simulink library "Lib_Turbo_Nozzle_TMATS"  (R2019b)
settings: Solver=ode45  StartTime=0.0  StopTime=10.0  RelTol=1e-3  EnableMultiTasking=on
undefined symbols (not defined in the file): stripchar_TMATS
libraries: Lib_Solve_DataOut_TMATS x1
Description:
  | Thomas Modules
settings Model: Creator=jwchapm2  LastModifiedBy=bhisma
settings DataIOCC: LimitDataPoints=on  SaveFormat=Array  ReturnWorkspaceOutputs=off
settings OptimizationCC: ExpressionDepthLimit=2147483647  LifeSpan=inf
settings DebuggingCC: UnderspecifiedInitializationDetection=Classic  MergeDetectMultiDrivingBlocksExec=none  SolverPrmCheckMsg=warning  StateNameClashWarn=warning  SFUnexpectedBacktrackingDiag=warning  SFNoUnconditionalDefaultTransitionDiag=warning  SFExecutionAtInitializationDiag=none  ArithmeticOperatorsInVariantConditions=warning
settings HardwareCC: ProdBitPerPointer=32  ProdBitPerSizeT=32  ProdBitPerPtrDiffT=32  ProdLargestAtomicFloat=None  ProdIntDivRoundTo=Undefined  ProdEndianess=Unspecified  ProdWordSize=32  ProdHWDeviceType=32-bit Generic
settings ModelReferenceCC: PropagateSignalLabelsOutOfModel=off
settings SFSimCC: SimUseLocalCustomCode=off  CustomCodeUndefinedFunction=UseInterfaceOnly
settings RTWCC: RTWUseLocalCustomCode=off
settings CodeAppCC: StateflowObjectComments=on
settings GRTTargetCC: TargetLangStandard=C89/C90 (ANSI)  GeneratePreprocessorConditionals=Disable all
settings ConfigComp: CovMetricSettings=dw  CovHtmlReporting=on  CovSaveCumulativeToWorkspaceVar=on  CovSaveSingleToWorkspaceVar=on  CovExternalEMLEnable=off

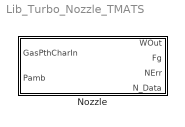
== system Lib_Turbo_Nozzle_TMATS ==
  Nozzle : Subsystem  mask(T-MATS: Nozzle Library Block){SWType_M=Convergent, N_TArea_M=110.7, N_EArea_M=110.7, N_FL_M=0.00, X_N_TtVec2_M=[300 10000], T_N_TGArray_M=[1 1], X_N_PEQPaVec_M=[0 10000], T_N_CdThArray_M=[1 1], T_N_CvArray_M=[1 1], CfgEn_M=off, T_N_CfgArray_M=[1 1], X_N_FARVec_M=[0; 0.0050; 0.0100; 0.0150; 0.0200; 0.0250; 0.0300], T_N_RtArray_M=[0.0686;    0.0686;    0.0686;    0.0686;    0.0686;    0.0686;    0.0686], Y_N_TtVec_M=[300 10000], T_N_MAP_gammaArray_M=[ 1.4 1.4 1.4 1.4 1.4 1.4 1.4; 1.4 1.4 1.4 1.4 1.4 1.4 1.4], iDesign_M=0, WDes_M=100, FVar_M=strcat('iDes_',stripchar_TMATS(gcb),'.bin')}
      mask prompts: SWType_M "SWType_M - Nozzle Type"; N_TArea_M "N_TArea_M - Nozzle Throat Area [in^2]"; N_EArea_M "N_EArea_M - Nozzle Exit Area [in^2], for CD nozzle only"; N_FL_M "N_FL_M - Flow Loss Across Nozzle [%]"; X_N_TtVec2_M "X_N_TtVec2_M - Nozzle Total Temperature Vector (X-axis for TG calc)(ax1)"; T_N_TGArray_M "T_N_TGArray_M - Nozzle Thermal Growth Array (TG = f(Tt))(ax1)"; X_N_PEQPaVec_M "X_N_PEQPaVec_M - Nozzle PE/Pa Vector (X-axis) (bx1)"; T_N_CdThArray_M "T_N_CdThArray_M - Nozzle CdTh Array, Blockage Factor [frac] (CdTh = f(PEQPa)) (bx1)"; T_N_CvArray_M "T_N_CvArray_M - Nozzle Velocity Coefficient Array (Cv = f(PEQPa)) (bx1)"; CfgEn_M "CfgEn_M - Enable Nozzle Thrust Coefficient"; T_N_CfgArray_M "T_N_CfgArray_M - Nozzle Thrust Coefficient Array (Cfg = f(PEQPa)) (bx1)"; X_N_FARVec_M "X_N_FARVec_M - Nozzle Fuel to Air Ratio Vector (X-axis) (cx1)"; T_N_RtArray_M "T_N_RtArray_M - Nozzle Gas Constant, R, Array (R = f(FAR))(cx1)"; Y_N_TtVec_M "Y_N_TtVec_M - Nozzle Total Temperature Vector (Y-axis for Gamma calc)(dx1)"; T_N_MAP_gammaArray_M "T_N_MAP_gammaArray_M - Nozzle Map Gamma Array (Gamma = f(Tt,FAR))(dxc)"; iDesign_M "iDesign_M - Design fork (0 - Enable iDes, 1 - Use iDes Ath, 2 - Use Input Ath)"; WDes_M "WDes_M - Design Flow [pps]"; FVar_M "FVar_M - File name for iDes Variables"
      mask help: This block simulates the performance of a nozzle using basic thermodynamic equations, properties, and table lookups.
      mask init:
      | if iDesign_M == 1
      |     P = load(FVar_M);
      |     N_TArea_M = P(1);
      |     N_EArea_M = P(2);
      | end
      mask Help: web(which('Turbo_TMATS_Noz.html'),'-helpbrowser')
      mask TypeOptions SWType_M: Convergent | Convergent-Divergent
      mask Callback SWType_M:
      | switch get_param(gcb,'iDesign_M')
      |     case ('2')
      |         switch get_param(gcb,'SWType_M')
      |             case ('Convergent')
      |                 MSK_SEC_Enables_Ides_TMATS(int16(1),[3],'G1')
      |             case ('Convergent-Divergent')
      |                 MSK_SEC_Enables_Ides_TMATS(int16(2),[3],'G1')
      |         end
      | end
      mask Callback CfgEn_M:
      | MSK_SEC_Enables_TMATS('CfgEn_M',[11],'en')
      | MSK_SEC_Enables_TMATS('CfgEn_M',[9],'dis')
      mask Callback iDesign_M:
      | switch get_param(gcb,'SWType_M')
      |     case ('Convergent-Divergent')
      |     MSK_SEC_Enables_Ides_TMATS('iDesign_M',[3],'G1')
      | end
      | 
      | MSK_SEC_Enables_Ides_TMATS('iDesign_M',[2],'G1')
      | MSK_SEC_Enables_Ides_TMATS('iDesign_M',[17],'G2')
      | MSK_SEC_Enables_Ides_TMATS('iDesign_M',[18],'G3')
      mask DialogControl ParameterTabVar0 Prompt: General
      mask DialogControl ParameterTabVar01 Prompt: GasProp
      mask DialogControl ParameterTabVar012 Prompt: iDesign

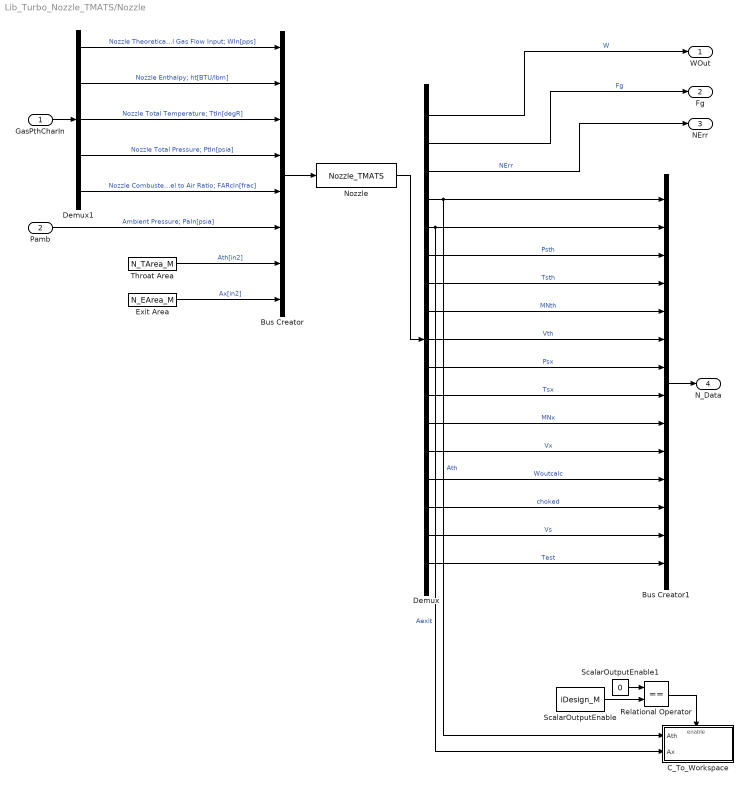
== system Lib_Turbo_Nozzle_TMATS/Nozzle ==
  GasPthCharIn : Inport
  Pamb : Inport  Port=2
  Bus Creator : BusCreator  Inputs=8
  Bus Creator1 : BusCreator  Inputs=14
  C_To_Workspace : Subsystem
  Demux : Demux  Outputs=17
  Demux1 : Demux  Outputs=5
  Exit Area : Constant  Value=N_EArea_M
  Nozzle : S-Function  FunctionName=Nozzle_TMATS  Parameters=SWType_M, N_FL_M, X_N_FARVec_M, T_N_RtArray_M, Y_N_TtVec_M, T_N_MAP_gammaArray_M, X_N_PEQPaVec_M, T_N_CdThArray_M, T_N_CvArray_M, T_N_CfgArray_M, T_N_TGArray_M, X_N_TtVec2_M, iDesign_M, WDes_M,CfgEn_M, gcs  SFunctionModules='pt2sc_TMATS sp2tc_TMATS t2hc_TMATS interp1Ac_TMATS interp2Ac_TMATS PcalcStat_TMATS functions_TMATS'  SFunctionDeploymentMode=off  EnableBusSupport=off
  Relational Operator : RelationalOperator  Operator===  OutDataTypeStr=boolean  RndMeth=Nearest
  ScalarOutputEnable : Constant  Value=iDesign_M
  ScalarOutputEnable1 : Constant  Value=0
  Throat Area : Constant  Value=N_TArea_M
  WOut : Outport
  Fg : Outport  Port=2
  NErr : Outport  Port=3
  N_Data : Outport  Port=4
  wires:
  Demux1/4 -> Bus Creator/4  "Nozzle Total Pressure; PtIn[psia]"
  Pamb/1 -> Bus Creator/6  "Ambient Pressure; PaIn[psia]"
  Bus Creator/1 -> Nozzle/1
  Demux/2 -> Fg/1  "Fg"
  Demux/1 -> WOut/1  "W"
  Nozzle/1 -> Demux/1
  Demux1/3 -> Bus Creator/3  "Nozzle Total Temperature; TtIn[degR]"
  Demux1/5 -> Bus Creator/5  "Nozzle Combusted Fuel to Air Ratio; FARcIn[frac]"
  Demux/5 -> Bus Creator1/2, C_To_Workspace/2(Ax)  "Aexit"
  GasPthCharIn/1 -> Demux1/1
  Demux1/1 -> Bus Creator/1  "Nozzle Theoretical Gas Flow Input; WIn[pps]"
  Demux/3 -> NErr/1  "NErr"
  Demux1/2 -> Bus Creator/2  "Nozzle Enthalpy; ht[BTU/lbm]"
  Demux/4 -> C_To_Workspace/1(Ath), Bus Creator1/1  "Ath"
  Bus Creator1/1 -> N_Data/1
  ScalarOutputEnable/1 -> Relational Operator/2
  ScalarOutputEnable1/1 -> Relational Operator/1
  Relational Operator/1 -> C_To_Workspace/Enable
  Throat Area/1 -> Bus Creator/7  "Ath[in2]"
  Exit Area/1 -> Bus Creator/8  "Ax[in2]"
  Demux/6 -> Bus Creator1/3  "Psth"
  Demux/14 -> Bus Creator1/11  "Woutcalc"
  Demux/13 -> Bus Creator1/10  "Vx"
  Demux/15 -> Bus Creator1/12  "choked"
  Demux/8 -> Bus Creator1/5  "MNth"
  Demux/9 -> Bus Creator1/6  "Vth"
  Demux/7 -> Bus Creator1/4  "Tsth"
  Demux/11 -> Bus Creator1/8  "Tsx"
  Demux/10 -> Bus Creator1/7  "Psx"
  Demux/12 -> Bus Creator1/9  "MNx"
  Demux/16 -> Bus Creator1/13  "Vs"
  Demux/17 -> Bus Creator1/14  "Test"

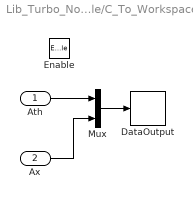
== system Lib_Turbo_Nozzle_TMATS/Nozzle/C_To_Workspace ==
  Ath : Inport
  Ax : Inport  Port=2
  Enable : EnablePort
  DataOutput : Lib_Solve_DataOut_TMATS/DataOutput  FVar_M=double(FVar_M)
  Mux : Mux  Inputs=2
  wires:
  Ath/1 -> Mux/1
  Ax/1 -> Mux/2
  Mux/1 -> DataOutput/1
